simulink library "LibraryForCodeGeneration"  (R2023b)
settings: Solver=VariableStepAuto  StartTime=0.0  StopTime=10.0  RelTol=1e-3
undefined symbols (not defined in the file or in its folder): DiscIntNeverNeededParam, Fnom_Grid, Ts, Ts_Control
libraries: $bdroot x18, simulink x2
settings Model: Creator=ZZY  LastModifiedBy=ZZY

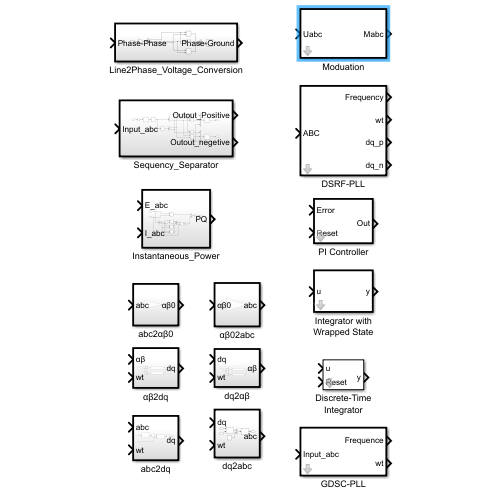
[thumbnail: Simulink's stored preview of the top-level diagram]
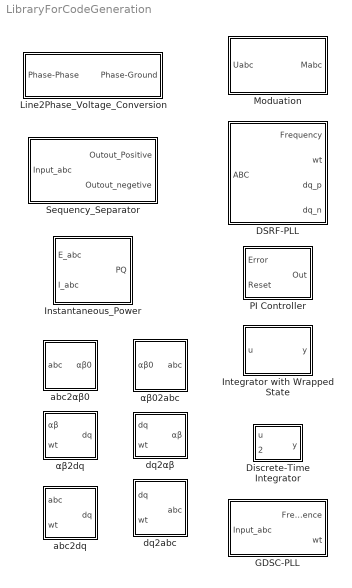
== system LibraryForCodeGeneration ==
  DSRF-PLL : Subsystem  TreatAsAtomicUnit=on  RTWFcnName=DSRF_PLL  mask{Ts=Ts_Control, Wc=2*pi*50*0.707, Wf=2*pi*50, Kp=2*pi*25*2*0.707, Ki=power(2*pi*25,2)}
      mask prompts: Ts "Sampling Time:"; Wc "Cut-off  frequency of the LPF(rad/s):"; Wf "Fundamental  frequency(rad/s):"
      settings: RTWFcnNameOpts=User specified
  Discrete-Time Integrator : Subsystem  mask{Ts=Ts}
      mask prompts: Ts "Sample time :"
  GDSC-PLL : Subsystem  TreatAsAtomicUnit=on  mask{Ts=Ts_Control, Fnom_Grid=50}
      mask prompts: Ts "Sample Time:"; Fnom_Grid "Rated Frequence of Grid:"
  Instantaneous_Power : Subsystem  TreatAsAtomicUnit=on  RTWFcnName=Instantaneous_Power
      settings: RTWFcnNameOpts=User specified
  Integrator with Wrapped State : Subsystem  TreatAsAtomicUnit=on  RTWFcnName=Wrapped_Integrator  VariantControl=Discrete  mask{WrappedStateUpperValue=0, WrappedStateLowerValue=0, Ts=-1}
      mask prompts: WrappedStateUpperValue "Wrapped state upper value:"; WrappedStateLowerValue "Wrapped state lower value:"; Ts "Sample time (-1 for inherited)"
      settings: RTWFcnNameOpts=User specified
  Line2Phase_Voltage_Conversion : Subsystem  TreatAsAtomicUnit=on  RTWFcnName=Line2Phase_Voltage_Conversion
      settings: RTWFcnNameOpts=User specified
  Moduation : Subsystem  TreatAsAtomicUnit=on  mask{Modulation=1}
      mask prompts: Modulation "Modulation Method(0->SPWM, 1->SVPWM):"
  PI Controller : Subsystem  TreatAsAtomicUnit=on  RTWFcnName=PI_Controller  mask{Kp=0, Ki=0, Ts=Ts_Control, Max=1, Min=-1}
      mask prompts: Kp "Proportional:"; Ki "Integral:"; Ts "Sampling Time  :"; Max "Up Limit of Saturation:"; Min "Low Limit of Saturation:"
      settings: RTWFcnNameOpts=User specified
  Sequency_Separator : Subsystem  TreatAsAtomicUnit=on  RTWFcnName=Sequency_Separator
      settings: RTWFcnNameOpts=User specified
  abc2dq : Subsystem  TreatAsAtomicUnit=on  RTWFcnName=abc2dq
      settings: RTWFcnNameOpts=User specified
  abc2αβ0 : Subsystem  TreatAsAtomicUnit=on  RTWFcnName=abc2AlphaBetaZero
      settings: RTWFcnNameOpts=User specified
  dq2abc : Subsystem  TreatAsAtomicUnit=on  RTWFcnName=dq2abc
      settings: RTWFcnNameOpts=User specified
  dq2αβ : Subsystem  TreatAsAtomicUnit=on  RTWFcnName=dq2AlphaBeta
      settings: RTWFcnNameOpts=User specified
  αβ02abc : Subsystem  TreatAsAtomicUnit=on  RTWFcnName=AlphaBetaZero2abc
      settings: RTWFcnNameOpts=User specified
  αβ2dq : Subsystem  TreatAsAtomicUnit=on  RTWFcnName=AlphaBeta2dq
      settings: RTWFcnNameOpts=User specified

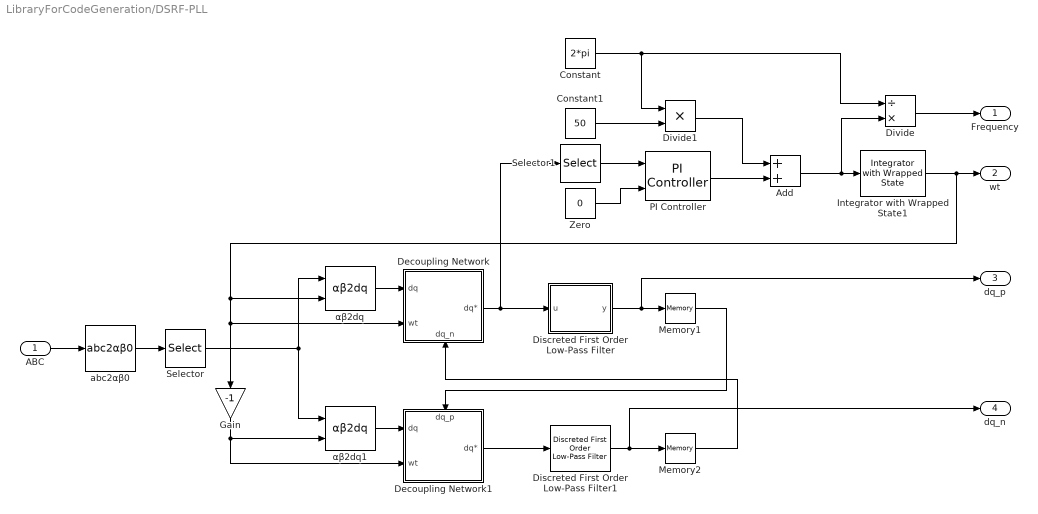
== system LibraryForCodeGeneration/DSRF-PLL ==
  ABC : Inport
  Add : Sum
  Constant : Constant  Value=2*pi  OutDataTypeStr=single  SampleTime=-1
  Constant1 : Constant  Value=50  OutDataTypeStr=Inherit: Inherit via back propagation  SampleTime=-1
  Decoupling Network : Subsystem
      settings: PortSchema="{\"entries\":[{\"content\":{\"sides\":[{\"content\":{\"connectorIds\":[\"In1\",\"In2\"]},\"type\":\"ConnectorPlacement.EquallySpacedRectSide\",\"uuid\":\"616b24e1-56e6-4614-ba2f-bd62e326c103\"},{\"content\":{\"connectorIds\":[\"Out1\"],\"side\":\"RIGHT\"},\"type\":\"ConnectorPlacement.EquallySpacedRectSide\",\"uuid\":\"d002ccc8-a8e9-4a33-b4ba-37ade36bc88e\"},{\"content\":{\"side\":\"TOP\"},\"type\":\"ConnectorPlacement.EquallySpacedRectSide\",\"uuid\":\"22e49a5d-b55b-4fa7-ad37-ecfc3ef17bd3\"},{\"content\":{\"connectorIds\":[\"In3\"],\"side\":\"BOTTOM\"},\"type\":\"ConnectorPlacement.EquallySpacedRectSide\",\"uuid\":\"7e8d98ba-e876-4857-9b05-7c0be2a1c9ed\"}]},\"type\":\"ConnectorPlacement.EquallySpacedConnector\",\"uuid\":\"40cd40bf-343a-4150-bffd-169ac481916a\"}],\"packageUris\":[\"http://schema.mathworks.com/mf0/Connector/R2020b\"],\"version\":\"1.0\"}"
  Decoupling Network1 : Subsystem
      settings: PortSchema="{\"entries\":[{\"content\":{\"sides\":[{\"content\":{\"connectorIds\":[\"In1\",\"In2\"]},\"type\":\"ConnectorPlacement.EquallySpacedRectSide\",\"uuid\":\"616b24e1-56e6-4614-ba2f-bd62e326c103\"},{\"content\":{\"connectorIds\":[\"Out1\"],\"side\":\"RIGHT\"},\"type\":\"ConnectorPlacement.EquallySpacedRectSide\",\"uuid\":\"d002ccc8-a8e9-4a33-b4ba-37ade36bc88e\"},{\"content\":{\"connectorIds\":[\"In3\"],\"side\":\"TOP\"},\"type\":\"ConnectorPlacement.EquallySpacedRectSide\",\"uuid\":\"22e49a5d-b55b-4fa7-ad37-ecfc3ef17bd3\"}]},\"type\":\"ConnectorPlacement.EquallySpacedConnector\",\"uuid\":\"40cd40bf-343a-4150-bffd-169ac481916a\"}],\"packageUris\":[\"http://schema.mathworks.com/mf0/Connector/R2020b\"],\"version\":\"1.0\"}"
  Discreted First Order Low-Pass Filter : Subsystem  TreatAsAtomicUnit=on  mask{Wc=Wc, Ts=Ts}
      mask prompts: Wc "Cut-off Frequency (rad):"; Ts "Sample time (-1 for inherited):"
  Discreted First Order Low-Pass Filter1 : $bdroot/DSRF-PLL/Discreted First Order Low-Pass Filter  Wc=Wc  Ts=Ts
  Divide : Product  Inputs=/*  OutDataTypeStr=Inherit: Inherit via back propagation
  Divide1 : Product  Inputs=**  OutDataTypeStr=Inherit: Inherit via back propagation
  Gain : Gain  Gain=-1
  Integrator with Wrapped State1 : $bdroot/Integrator with Wrapped State  VariantControl=Discrete  WrappedStateUpperValue=2*pi  WrappedStateLowerValue=0  Ts=Ts
  Memory1 : Memory  InheritSampleTime=on
  Memory2 : Memory  InheritSampleTime=on
  PI Controller : $bdroot/PI Controller  Kp=Kp  Ki=Ki  Ts=Ts  Max=2*Wf  Min=-2*Wf
  Selector : Selector  InputPortWidth=3  IndexOptions=Index vector (dialog)  Indices=[1 2]  OutputSizes=1
  Selector1 : Selector  InputPortWidth=2  IndexOptions=Index vector (dialog)  Indices=[2]  OutputSizes=1
  Zero : Constant  Value=0  OutDataTypeStr=boolean  SampleTime=-1
  abc2αβ0 : $bdroot/abc2αβ0  SystemSampleTime=-1  VariantActivationTime=update diagram  AllowFlexibleInterface=on  Latency=0  AutoFrameSizeCalculation=off
  αβ2dq : $bdroot/αβ2dq  SystemSampleTime=-1  VariantActivationTime=update diagram  AllowFlexibleInterface=on  Latency=0  AutoFrameSizeCalculation=off
  αβ2dq1 : $bdroot/αβ2dq  SystemSampleTime=-1  VariantActivationTime=update diagram  AllowFlexibleInterface=on  Latency=0  AutoFrameSizeCalculation=off
  Frequency : Outport
  wt : Outport  Port=2
  dq_p : Outport  Port=3
  dq_n : Outport  Port=4
  wires:
  Decoupling Network/1(dq*) -> Discreted First Order Low-Pass Filter/1(u), Selector1/1
  Selector/1 -> αβ2dq1/1, αβ2dq/1
  Add/1 -> Integrator with Wrapped State1/1, Divide/2
  ABC/1 -> abc2αβ0/1
  abc2αβ0/1 -> Selector/1
  Gain/1 -> Decoupling Network1/2(wt), αβ2dq1/2
  Constant/1 -> Divide/1, Divide1/1
  Decoupling Network1/1(dq*) -> Discreted First Order Low-Pass Filter1/1
  αβ2dq1/1 -> Decoupling Network1/1(dq)
  Selector1/1 -> PI Controller/1
  αβ2dq/1 -> Decoupling Network/1(dq)
  Divide/1 -> Frequency/1
  Discreted First Order Low-Pass Filter/1(y) -> dq_p/1, Memory1/1
  Integrator with Wrapped State1/1 -> Decoupling Network/2(wt), Gain/1, αβ2dq/2, wt/1
  PI Controller/1 -> Add/2
  Constant1/1 -> Divide1/2
  Divide1/1 -> Add/1
  Zero/1 -> PI Controller/2
  Memory1/1 -> Decoupling Network1/3(dq_p)
  Memory2/1 -> Decoupling Network/3(dq_n)
  Discreted First Order Low-Pass Filter1/1 -> dq_n/1, Memory2/1

== system LibraryForCodeGeneration/Discrete-Time Integrator ==
  u : Inport
  Reset : Inport  Port=2
  Add3 : Sum  Inputs=|++
  Delay : Delay  DelayLength=1  ExternalReset=Rising  SampleTime=Ts
      settings: InputPortMap=u0,r5
  Gain2 : Gain  Gain=Ts
  y : Outport
  wires:
  Add3/1 -> Delay/1
  u/1 -> Add3/1
  Gain2/1 -> y/1
  Reset/1 -> Delay/2
  Delay/1 -> Add3/2, Gain2/1

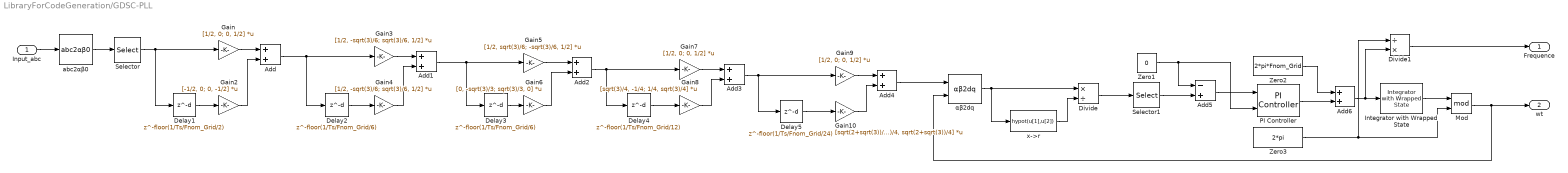
== system LibraryForCodeGeneration/GDSC-PLL ==
  Input_abc : Inport
  Add{,1..4,6} (6 alike) : Sum
  Add5 : Sum  Inputs=-+
  Delay1 : Delay  DelayLength=floor(1/Ts/Fnom_Grid/2)  SampleTime=Ts
  Delay2 : Delay  DelayLength=floor(1/Ts/Fnom_Grid/6)  SampleTime=Ts
  Delay3 : Delay  DelayLength=floor(1/Ts/Fnom_Grid/6)  SampleTime=Ts
  Delay4 : Delay  DelayLength=floor(1/Ts/Fnom_Grid/12)  SampleTime=Ts
  Delay5 : Delay  DelayLength=floor(1/Ts/Fnom_Grid/24)  SampleTime=Ts
  Divide : Product  Inputs=*/
  Divide1 : Product  Inputs=/*
  Gain : Gain  Gain=[1/2, 0; 0, 1/2]  Multiplication=Matrix(K*u)
  Gain10 : Gain  Gain=[sqrt(2+sqrt(3))/4, -sqrt(2-sqrt(3))/4; sqrt(2-sqrt(3))/4, sqrt(2+sqrt(3))/4]  Multiplication=Matrix(K*u)
  Gain2 : Gain  Gain=[-1/2, 0; 0, -1/2]  Multiplication=Matrix(K*u)
  Gain3 : Gain  Gain=[1/2, -sqrt(3)/6; sqrt(3)/6, 1/2]  Multiplication=Matrix(K*u)
  Gain4 : Gain  Gain=[1/2, -sqrt(3)/6; sqrt(3)/6, 1/2]  Multiplication=Matrix(K*u)
  Gain5 : Gain  Gain=[1/2, sqrt(3)/6; -sqrt(3)/6, 1/2]  Multiplication=Matrix(K*u)
  Gain6 : Gain  Gain=[0, -sqrt(3)/3; sqrt(3)/3, 0]  Multiplication=Matrix(K*u)
  Gain7 : Gain  Gain=[1/2, 0; 0, 1/2]  Multiplication=Matrix(K*u)
  Gain8 : Gain  Gain=[sqrt(3)/4, -1/4; 1/4, sqrt(3)/4]  Multiplication=Matrix(K*u)
  Gain9 : Gain  Gain=[1/2, 0; 0, 1/2]  Multiplication=Matrix(K*u)
  Integrator with Wrapped State : $bdroot/Integrator with Wrapped State  VariantControl=Discrete  WrappedStateUpperValue=2*pi*1000  WrappedStateLowerValue=0  Ts=Ts
  Mod : Math  Operator=mod
  PI Controller : $bdroot/PI Controller  Kp=0.707*sqrt(4*power(2*pi*100,2))  Ki=power(2*pi*100,2)  Ts=Ts  Max=2*pi*100  Min=-2*pi*100
  Selector : Selector  InputPortWidth=3  IndexOptions=Index vector (dialog)  Indices=[1 2]  OutputSizes=1
  Selector1 : Selector  InputPortWidth=2  IndexOptions=Index vector (dialog)  Indices=[2]  OutputSizes=1
  Zero1 : Constant  Value=0  OutDataTypeStr=Inherit: Inherit via back propagation
  Zero2 : Constant  Value=2*pi*Fnom_Grid  OutDataTypeStr=Inherit: Inherit via back propagation
  Zero3 : Constant  Value=2*pi  OutDataTypeStr=Inherit: Inherit via back propagation
  abc2αβ0 : $bdroot/abc2αβ0  SystemSampleTime=-1  VariantActivationTime=update diagram  AllowFlexibleInterface=on  Latency=0  AutoFrameSizeCalculation=off
  x->r : Fcn  Expr=hypot(u[1],u[2])
  αβ2dq : $bdroot/αβ2dq  SystemSampleTime=-1  VariantActivationTime=update diagram  AllowFlexibleInterface=on  Latency=0  AutoFrameSizeCalculation=off
  Frequence : Outport
  wt : Outport  Port=2
  wires:
  Delay1/1 -> Gain2/1
  Selector/1 -> Gain/1, Delay1/1
  abc2αβ0/1 -> Selector/1
  Input_abc/1 -> abc2αβ0/1
  Gain/1 -> Add/1
  Gain2/1 -> Add/2
  Add/1 -> Delay2/1, Gain3/1
  Delay2/1 -> Gain4/1
  Gain3/1 -> Add1/1
  Gain4/1 -> Add1/2
  Add1/1 -> Gain5/1, Delay3/1
  Delay3/1 -> Gain6/1
  Gain5/1 -> Add2/1
  Gain6/1 -> Add2/2
  Delay4/1 -> Gain8/1
  Add2/1 -> Delay4/1, Gain7/1
  Add3/1 -> Gain9/1, Delay5/1
  Delay5/1 -> Gain10/1
  Gain7/1 -> Add3/1
  Gain9/1 -> Add4/1
  Gain8/1 -> Add3/2
  Gain10/1 -> Add4/2
  αβ2dq/1 -> Divide/1, x->r/1
  x->r/1 -> Divide/2
  Divide/1 -> Selector1/1
  Selector1/1 -> Add5/2
  Zero1/1 -> Add5/1, PI Controller/2
  Add5/1 -> PI Controller/1
  PI Controller/1 -> Add6/2
  Zero2/1 -> Add6/1
  Add6/1 -> Integrator with Wrapped State/1, Divide1/2
  Mod/1 -> αβ2dq/2, wt/1
  Divide1/1 -> Frequence/1
  Zero3/1 -> Mod/2, Divide1/1
  Add4/1 -> αβ2dq/1
  Integrator with Wrapped State/1 -> Mod/1

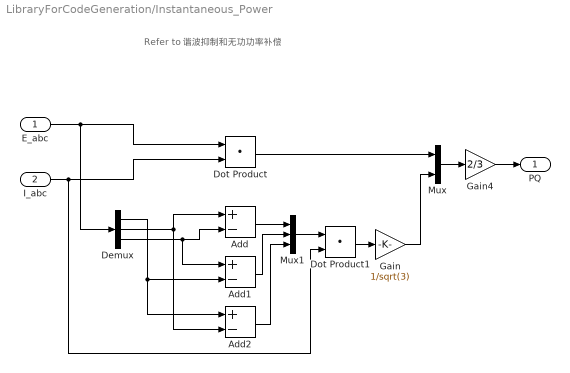
== system LibraryForCodeGeneration/Instantaneous_Power ==
  note: Refer to 谐波抑制和无功功率补偿
  E_abc : Inport
  I_abc : Inport  Port=2
  Add : Sum  Inputs=+-
  Add1 : Sum  Inputs=+-
  Add2 : Sum  Inputs=+-
  Demux : Demux  Outputs=3
  Dot Product : DotProduct  OutDataTypeStr=Inherit: Inherit via internal rule
  Dot Product1 : DotProduct  OutDataTypeStr=Inherit: Inherit via internal rule
  Gain : Gain  Gain=1/sqrt(3)
  Gain4 : Gain  Gain=2/3
  Mux : Mux  Inputs=2
  Mux1 : Mux  Inputs=3
  PQ : Outport
  wires:
  E_abc/1 -> Demux/1, Dot Product/1
  I_abc/1 -> Dot Product/2, Dot Product1/2
  Mux/1 -> Gain4/1
  Dot Product/1 -> Mux/1
  Demux/2 -> Add2/2, Add/1
  Demux/3 -> Add1/1, Add/2
  Demux/1 -> Add2/1, Add1/2
  Add/1 -> Mux1/1
  Add1/1 -> Mux1/2
  Add2/1 -> Mux1/3
  Mux1/1 -> Dot Product1/1
  Dot Product1/1 -> Gain/1
  Gain/1 -> Mux/2
  Gain4/1 -> PQ/1

== system LibraryForCodeGeneration/Integrator with Wrapped State ==
  u : Inport
  Compare To Constant : simulink/Logic and Bit Operations/Compare To Constant  relop=<  const=WrappedStateLowerValue  OutDataTypeStr=boolean
  Compare To Constant1 : simulink/Logic and Bit Operations/Compare To Constant  relop=>=  const=WrappedStateUpperValue  OutDataTypeStr=boolean
  Integrator : DiscreteIntegrator  ExternalReset=sampled level  SampleTime=Ts  ShowStatePort=on  ICPrevOutput=DiscIntNeverNeededParam  ICPrevScaledInput=DiscIntNeverNeededParam
  Logical Operator : Logic  Operator=OR  AllPortsSameDT=off  OutDataTypeStr=boolean
  y : Outport  VectorParamsAs1DForOutWhenUnconnected=off
  wires:
  Logical Operator/1 -> Integrator/2
  u/1 -> Integrator/1
  Compare To Constant1/1 -> Logical Operator/2
  Integrator/State -> Compare To Constant/1, Compare To Constant1/1
  Integrator/1 -> y/1
  Compare To Constant/1 -> Logical Operator/1

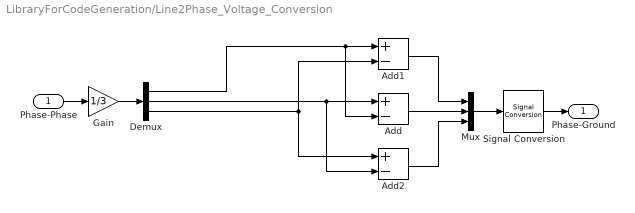
== system LibraryForCodeGeneration/Line2Phase_Voltage_Conversion ==
  Phase-Phase : Inport
  Add : Sum  Inputs=+-
  Add1 : Sum  Inputs=+-
  Add2 : Sum  Inputs=+-
  Demux : Demux  Outputs=3
  Gain : Gain  Gain=1/3
  Mux : Mux  Inputs=3
  Signal Conversion : SignalConversion  OverrideOpt=off
  Phase-Ground : Outport
  wires:
  Phase-Phase/1 -> Gain/1
  Gain/1 -> Demux/1
  Mux/1 -> Signal Conversion/1
  Add/1 -> Mux/2
  Add1/1 -> Mux/1
  Add2/1 -> Mux/3
  Signal Conversion/1 -> Phase-Ground/1
  Demux/1 -> Add/2, Add1/1
  Demux/3 -> Add2/1, Add1/2
  Demux/2 -> Add2/2, Add/1

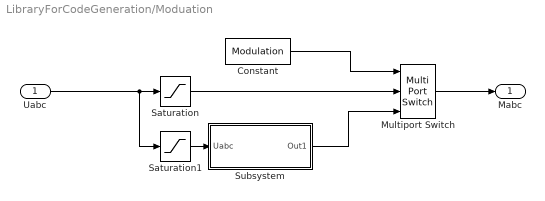
== system LibraryForCodeGeneration/Moduation ==
  Uabc : Inport
  Constant : Constant  Value=Modulation  OutDataTypeStr=uint16  SampleTime=Ts_Control
  Multiport Switch : MultiPortSwitch  DataPortOrder=Zero-based contiguous  Inputs=2  zeroidx=on  SaturateOnIntegerOverflow=off  InputSameDT=off
  Saturation : Saturate  UpperLimit=1  LowerLimit=-1
  Saturation1 : Saturate  UpperLimit=1.15  LowerLimit=-1.15
  Subsystem : Subsystem
  Mabc : Outport
  wires:
  Multiport Switch/1 -> Mabc/1
  Constant/1 -> Multiport Switch/1
  Subsystem/1(Out1) -> Multiport Switch/3
  Uabc/1 -> Saturation1/1, Saturation/1
  Saturation1/1 -> Subsystem/1(Uabc)
  Saturation/1 -> Multiport Switch/2

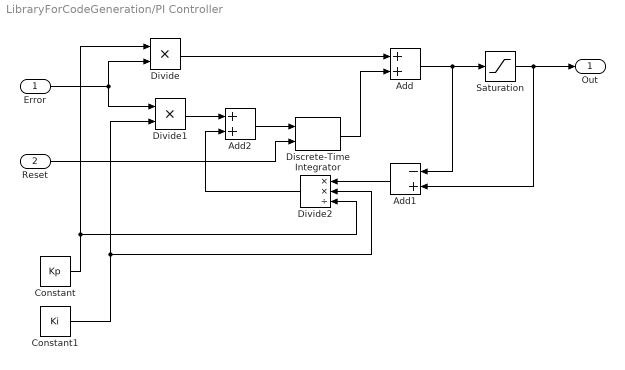
== system LibraryForCodeGeneration/PI Controller ==
  Error : Inport
  Reset : Inport  Port=2  OutDataTypeStr=boolean
  Add : Sum
  Add1 : Sum  Inputs=-+
  Add2 : Sum
  Constant : Constant  Value=Kp  OutDataTypeStr=Inherit: Inherit via back propagation  SampleTime=-1
  Constant1 : Constant  Value=Ki  OutDataTypeStr=Inherit: Inherit via back propagation  SampleTime=-1
  Discrete-Time Integrator : $bdroot/Discrete-Time Integrator  Ts=Ts
  Divide : Product  Inputs=**
  Divide1 : Product  Inputs=**
  Divide2 : Product  Inputs=**/
  Saturation : Saturate  UpperLimit=Max  LowerLimit=Min
  Out : Outport
  wires:
  Divide1/1 -> Add2/1
  Error/1 -> Divide1/1, Divide/2
  Divide/1 -> Add/1
  Saturation/1 -> Out/1, Add1/2
  Constant/1 -> Divide2/3, Divide/1
  Add2/1 -> Discrete-Time Integrator/1
  Add/1 -> Add1/1, Saturation/1
  Reset/1 -> Discrete-Time Integrator/2
  Add1/1 -> Divide2/1
  Discrete-Time Integrator/1 -> Add/2
  Constant1/1 -> Divide1/2, Divide2/2
  Divide2/1 -> Add2/2

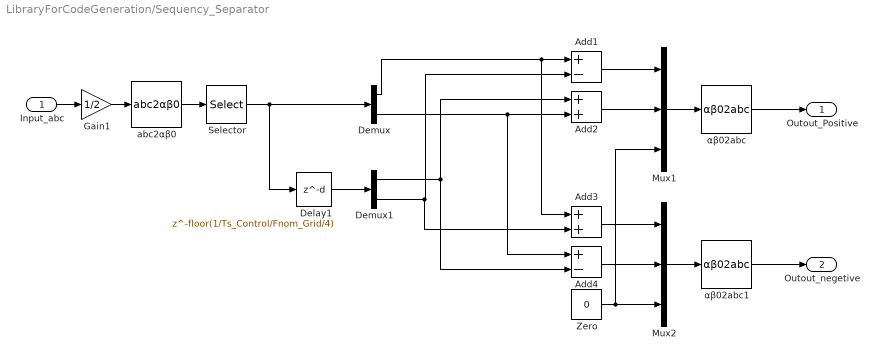
== system LibraryForCodeGeneration/Sequency_Separator ==
  Input_abc : Inport
  Add1 : Sum  Inputs=+-
  Add2 : Sum
  Add3 : Sum
  Add4 : Sum  Inputs=+-
  Delay1 : Delay  DelayLength=floor(1/Ts_Control/Fnom_Grid/4)  SampleTime=Ts_Control
  Demux : Demux  Outputs=2
  Demux1 : Demux  Outputs=2
  Gain1 : Gain  Gain=1/2
  Mux1 : Mux  Inputs=3
  Mux2 : Mux  Inputs=3
  Selector : Selector  InputPortWidth=3  IndexOptions=Index vector (dialog)  Indices=[1 2]  OutputSizes=1
  Zero : Constant  Value=0  OutDataTypeStr=Inherit: Inherit via back propagation
  abc2αβ0 : $bdroot/abc2αβ0  SystemSampleTime=-1  VariantActivationTime=update diagram  AllowFlexibleInterface=on  Latency=0  AutoFrameSizeCalculation=off
  αβ02abc : $bdroot/αβ02abc  SystemSampleTime=-1  VariantActivationTime=update diagram  AllowFlexibleInterface=on  Latency=0  AutoFrameSizeCalculation=off
  αβ02abc1 : $bdroot/αβ02abc  SystemSampleTime=-1  VariantActivationTime=update diagram  AllowFlexibleInterface=on  Latency=0  AutoFrameSizeCalculation=off
  Outout_Positive : Outport
  Outout_negetive : Outport  Port=2
  wires:
  Add3/1 -> Mux2/1
  Delay1/1 -> Demux1/1
  αβ02abc/1 -> Outout_Positive/1
  Mux2/1 -> αβ02abc1/1
  Mux1/1 -> αβ02abc/1
  Zero/1 -> Mux1/3, Mux2/3
  abc2αβ0/1 -> Selector/1
  Selector/1 -> Delay1/1, Demux/1
  Add4/1 -> Mux2/2
  Demux/1 -> Add3/1, Add1/1
  Demux1/1 -> Add4/2, Add2/1
  Add1/1 -> Mux1/1
  Gain1/1 -> abc2αβ0/1
  Demux1/2 -> Add3/2, Add1/2
  Demux/2 -> Add4/1, Add2/2
  Add2/1 -> Mux1/2
  Input_abc/1 -> Gain1/1
  αβ02abc1/1 -> Outout_negetive/1

== system LibraryForCodeGeneration/abc2dq ==
  abc : Inport
  wt : Inport  Port=2
  Selector : Selector  InputPortWidth=3  IndexOptions=Index vector (dialog)  Indices=[1 2]  OutputSizes=1
  Signal Conversion : SignalConversion  OverrideOpt=off
  abc2αβ0 : $bdroot/abc2αβ0  SystemSampleTime=-1  VariantActivationTime=update diagram  AllowFlexibleInterface=on  Latency=0  AutoFrameSizeCalculation=off
  αβ2dq : $bdroot/αβ2dq  SystemSampleTime=-1  VariantActivationTime=update diagram  AllowFlexibleInterface=on  Latency=0  AutoFrameSizeCalculation=off
  dq : Outport
  wires:
  wt/1 -> αβ2dq/2
  Selector/1 -> αβ2dq/1
  abc2αβ0/1 -> Selector/1
  αβ2dq/1 -> Signal Conversion/1
  abc/1 -> abc2αβ0/1
  Signal Conversion/1 -> dq/1

== system LibraryForCodeGeneration/abc2αβ0 ==
  abc : Inport  PortDimensions=3
  Gain1 : Gain  Gain=2/3  SaturateOnIntegerOverflow=on  OutDataTypeStr=Inherit: Same as input  ParamDataTypeStr=Inherit: Same as input
  Gain3 : Gain  Gain="[ 1   -1/2   -1/2; 0   sqrt(3)/2   -sqrt(3)/2; 1/2  1/2  1/2 ]"  Multiplication=Matrix(K*u)  SaturateOnIntegerOverflow=on  OutDataTypeStr=Inherit: Same as input  ParamDataTypeStr=Inherit: Same as input
  αβ0 : Outport  VectorParamsAs1DForOutWhenUnconnected=off
  wires:
  abc/1 -> Gain3/1
  Gain1/1 -> αβ0/1
  Gain3/1 -> Gain1/1

== system LibraryForCodeGeneration/dq2abc ==
  dq : Inport
  wt : Inport  Port=2
  Constant : Constant  Value=0  OutDataTypeStr=Inherit: Inherit via back propagation
  Mux : Mux  Inputs=2
  dq2αβ0 : $bdroot/dq2αβ  SystemSampleTime=-1  VariantActivationTime=update diagram  AllowFlexibleInterface=on  Latency=0  AutoFrameSizeCalculation=off
  αβ02abc : $bdroot/αβ02abc  SystemSampleTime=-1  VariantActivationTime=update diagram  AllowFlexibleInterface=on  Latency=0  AutoFrameSizeCalculation=off
  abc : Outport
  wires:
  Mux/1 -> αβ02abc/1
  dq2αβ0/1 -> Mux/1
  dq/1 -> dq2αβ0/1
  wt/1 -> dq2αβ0/2
  αβ02abc/1 -> abc/1
  Constant/1 -> Mux/2

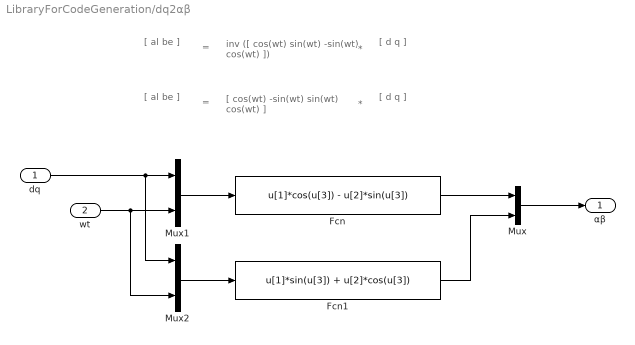
== system LibraryForCodeGeneration/dq2αβ ==
  note: =
  note: [  al
      |     be  ]
  note: [  al
      |     be  ]
  note: *
  note: [ d
      |    q ]
  note: [ d
      |    q ]
  note: inv ([  cos(wt)   sin(wt)
      |    -sin(wt)    cos(wt)   ])
  note: [  cos(wt)   -sin(wt)
      |    sin(wt)    cos(wt)   ]
  note: *
  note: =
  dq : Inport  PortDimensions=2
  wt : Inport  Port=2  PortDimensions=1
  Fcn : Fcn  Expr=u[1]*cos(u[3]) - u[2]*sin(u[3])
  Fcn1 : Fcn  Expr=u[1]*sin(u[3]) + u[2]*cos(u[3])
  Mux : Mux  Inputs=2
  Mux1 : Mux  Inputs=[2 1]
  Mux2 : Mux  Inputs=[2 1]
  αβ : Outport  InitialOutput=[0,0]  VectorParamsAs1DForOutWhenUnconnected=off
  wires:
  Fcn/1 -> Mux/1
  wt/1 -> Mux2/2, Mux1/2
  Mux1/1 -> Fcn/1
  dq/1 -> Mux2/1, Mux1/1
  Fcn1/1 -> Mux/2
  Mux/1 -> αβ/1
  Mux2/1 -> Fcn1/1

== system LibraryForCodeGeneration/αβ02abc ==
  αβ0 : Inport
  Gain3 : Gain  Gain="[ 1   0   1; -1/2  sqrt(3)/2   1; -1/2  -sqrt(3)/2  1 ]"  Multiplication=Matrix(K*u) (u vector)  SaturateOnIntegerOverflow=on  OutDataTypeStr=Inherit: Same as input  ParamDataTypeStr=Inherit: Same as input
  abc : Outport
  wires:
  Gain3/1 -> abc/1
  αβ0/1 -> Gain3/1

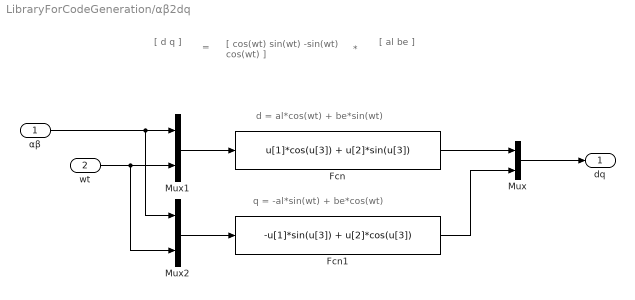
== system LibraryForCodeGeneration/αβ2dq ==
  note: [  al
      |     be  ]
  note: =
  note: [  cos(wt)   sin(wt)
      |    -sin(wt)    cos(wt)   ]
  note: q = -al*sin(wt) + be*cos(wt)
  note: *
  note: d = al*cos(wt) + be*sin(wt)
  note: [ d
      |    q ]
  αβ : Inport  PortDimensions=2
  wt : Inport  Port=2  PortDimensions=1
  Fcn : Fcn  Expr=u[1]*cos(u[3]) + u[2]*sin(u[3])
  Fcn1 : Fcn  Expr=-u[1]*sin(u[3]) + u[2]*cos(u[3])
  Mux : Mux  Inputs=2
  Mux1 : Mux  Inputs=[2 1]
  Mux2 : Mux  Inputs=[2 1]
  dq : Outport  InitialOutput=[0,0]  VectorParamsAs1DForOutWhenUnconnected=off
  wires:
  Mux2/1 -> Fcn1/1
  wt/1 -> Mux1/2, Mux2/2
  Mux/1 -> dq/1
  Mux1/1 -> Fcn/1
  Fcn/1 -> Mux/1
  αβ/1 -> Mux1/1, Mux2/1
  Fcn1/1 -> Mux/2

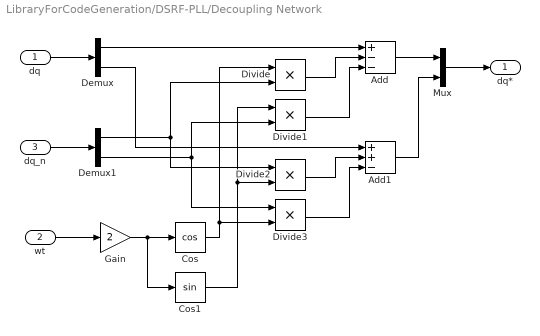
== system LibraryForCodeGeneration/DSRF-PLL/Decoupling Network ==
  dq : Inport
  wt : Inport  Port=2
  dq_n : Inport  Port=3
  Add : Sum  Inputs=+--  OutDataTypeStr=Inherit: Same as first input
  Add1 : Sum  Inputs=++-  OutDataTypeStr=Inherit: Same as first input
  Cos : Trigonometry  Operator=cos
  Cos1 : Trigonometry
  Demux : Demux  Outputs=2
  Demux1 : Demux  Outputs=2
  Divide{,1..3} (4 alike) : Product  Inputs=**
  Gain : Gain  Gain=2
  Mux : Mux  Inputs=2
  dq* : Outport
  wires:
  wt/1 -> Gain/1
  dq/1 -> Demux/1
  Gain/1 -> Cos1/1, Cos/1
  Demux/1 -> Add/1
  Divide/1 -> Add/2
  Cos/1 -> Divide3/2, Divide/1
  dq_n/1 -> Demux1/1
  Demux1/1 -> Divide2/1, Divide/2
  Cos1/1 -> Divide2/2, Divide1/1
  Demux1/2 -> Divide3/1, Divide1/2
  Divide1/1 -> Add/3
  Add/1 -> Mux/1
  Mux/1 -> dq*/1
  Divide2/1 -> Add1/2
  Divide3/1 -> Add1/3
  Demux/2 -> Add1/1
  Add1/1 -> Mux/2

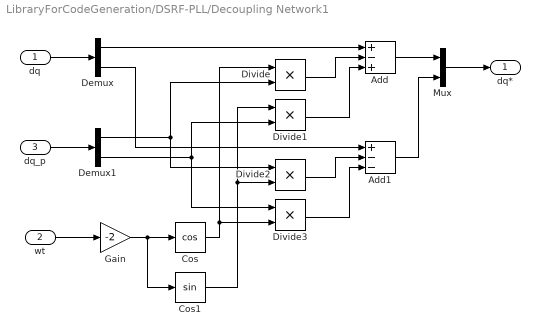
== system LibraryForCodeGeneration/DSRF-PLL/Decoupling Network1 ==
  dq : Inport
  wt : Inport  Port=2
  dq_p : Inport  Port=3
  Add : Sum  Inputs=+-+  OutDataTypeStr=Inherit: Same as first input
  Add1 : Sum  Inputs=+--  OutDataTypeStr=Inherit: Same as first input
  Cos : Trigonometry  Operator=cos
  Cos1 : Trigonometry
  Demux : Demux  Outputs=2
  Demux1 : Demux  Outputs=2
  Divide{,1..3} (4 alike) : Product  Inputs=**
  Gain : Gain  Gain=-2
  Mux : Mux  Inputs=2
  dq* : Outport
  wires:
  Divide/1 -> Add/2
  wt/1 -> Gain/1
  Demux/2 -> Add1/1
  Divide3/1 -> Add1/3
  Divide2/1 -> Add1/2
  Add/1 -> Mux/1
  Add1/1 -> Mux/2
  Divide1/1 -> Add/3
  dq_p/1 -> Demux1/1
  Demux1/1 -> Divide2/1, Divide/2
  Cos/1 -> Divide3/2, Divide/1
  Demux1/2 -> Divide3/1, Divide1/2
  dq/1 -> Demux/1
  Cos1/1 -> Divide2/2, Divide1/1
  Demux/1 -> Add/1
  Gain/1 -> Cos1/1, Cos/1
  Mux/1 -> dq*/1

== system LibraryForCodeGeneration/DSRF-PLL/Discreted First Order Low-Pass Filter ==
  u : Inport
  Add3 : Sum  Inputs=|+-
  Delay : Delay  DelayLength=1
  Gain1 : Gain  Gain=Ts*Wc-1
  Gain2 : Gain  Gain=Ts*Wc
  y : Outport
  wires:
  Add3/1 -> Delay/1
  u/1 -> Add3/1
  Gain1/1 -> Add3/2
  Delay/1 -> Gain2/1, Gain1/1
  Gain2/1 -> y/1

== system LibraryForCodeGeneration/Moduation/Subsystem ==
  Uabc : Inport
  Add : Sum
  Add1 : Sum  Inputs=+-
  Gain : Gain  Gain=1/2
  Max : MinMax  Function=max
  Max1 : MinMax
  Out1 : Outport
  wires:
  Uabc/1 -> Add1/1, Max1/1, Max/1
  Max/1 -> Add/1
  Max1/1 -> Add/2
  Add/1 -> Gain/1
  Add1/1 -> Out1/1
  Gain/1 -> Add1/2
